simulink model "PositionControlServoValve"  (R2024b)
settings: Solver=daessc  StartTime=0.0  StopTime=4  MaxStep=0.08  RelTol=1e-3  AbsTol=1e-3
PreLoadFcn:
  | PositionControlServoValveInput
values from neighbouring files (symbols this model uses):
  closePosition = 3e-4    (= 0.0003)    [PositionControlServoValveInput.m]
  dampCoeff = 1e-1    (= 0.1)    [PositionControlServoValveInput.m]
  flapperLength = 5e-3    (= 0.005)    [PositionControlServoValveInput.m]
  flapperRotAngle = 3.4928    [PositionControlServoValveInput.m]
  kii = 0.002    [PositionControlServoValveInput.m]
  kip = 0.004    [PositionControlServoValveInput.m]
  kpi = 600    [PositionControlServoValveInput.m]
  kpp = 160    [PositionControlServoValveInput.m]
  kvi = 10    [PositionControlServoValveInput.m]
  kvp = 200    [PositionControlServoValveInput.m]
  motorC = 1    [PositionControlServoValveInput.m]
  motorDampCoeff = 1e-3    (= 0.001)    [PositionControlServoValveInput.m]
  motorR = 750    [PositionControlServoValveInput.m]
  nozCrossSectArea = (pi/4)*(1.6e-3^2)    (= 2.0106192983e-06)    [PositionControlServoValveInput.m]
  overlap = 0.1    [PositionControlServoValveInput.m]
undefined symbols (not defined in the file or in its folder): smiData, X, Y, Z
libraries: fl_lib x174, sm_lib x50, SimscapeFluids_lib x43, nesl_utility x13
(part 4 of 5)

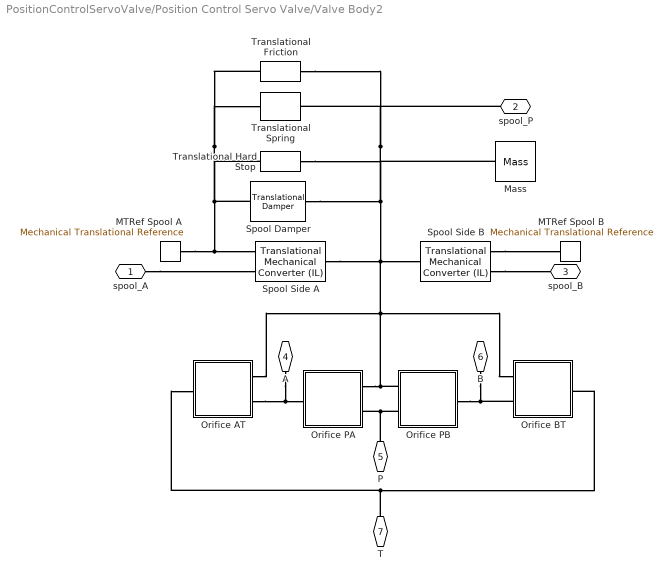
== system PositionControlServoValve/Position Control Servo Valve/Valve Body2 ==
  MTRef Spool A : fl_lib/Mechanical/Translational Elements/Mechanical Translational Reference  Tag=Factory Generic
  MTRef Spool B : fl_lib/Mechanical/Translational Elements/Mechanical Translational Reference  Tag=Factory Generic
  Mass : fl_lib/Mechanical/Translational Elements/Mass  mass=spoolMass kg  num_ports=foundation.enum.numPorts2.one  v_specify=off  v_priority=High  v=0 m/s  v_nominal_specify=off  v_nominal_value=1  v_nominal_unit=m/s  f_specify=off  f_priority=None  f=0 N  f_nominal_specify=off  f_nominal_value=1  f_nominal_unit=N
  Orifice AT : Subsystem  Tag=PublishSubsystem
  Orifice BT : Subsystem
  Orifice PA : Subsystem
  Orifice PB : Subsystem
  Spool Damper : fl_lib/Mechanical/Translational Elements/Translational Damper  Tag=Factory Generic  D=dampCoeff N/(m/s)  v_specify=off  v_priority=High  v=0 m/s  v_nominal_specify=off  v_nominal_value=1  v_nominal_unit=m/s  f_specify=off  f_priority=High  f=0 N  f_nominal_specify=off  f_nominal_value=1  f_nominal_unit=N
  Spool Side A : fl_lib/Isothermal Liquid/Elements/Translational Mechanical Converter (IL)  Tag=Factory Generic  mech_orientation=foundation.enum.MechOrientationTranslational.Positive  displacement_spec=foundation.enum.DisplacementSpec.Calculate  x0=0 m  interface_area=spoolArea mm^2  dead_volume=deadVol m^3  pressure_spec=foundation.enum.pressure_spec.atmospheric  environment_pressure=0.101325 MPa  dynamic_compressibility=simscape.enum.onoff.on  p0=pInitLeftChamber MPa
      settings: InternalSimscapePortConfiguration="{\"Bottom\":[],\"Left\":[{\"id\":\"A\",\"label\":\"A\",\"type\":\"foundation.isothermal_liquid.isothermal_liquid\"},{\"id\":\"C\",\"label\":\"C\",\"type\":\"foundation.mechanical.translational.translational\"}],\"Right\":[{\"id\":\"R\",\"label\":\"R\",\"type\":\"foundation.mechanical.translational.translational\"}],\"Top\":[]}"
  Spool Side B : fl_lib/Isothermal Liquid/Elements/Translational Mechanical Converter (IL)  Tag=Factory Generic  mech_orientation=foundation.enum.MechOrientationTranslational.Negative  displacement_spec=foundation.enum.DisplacementSpec.Calculate  x0=0 m  interface_area=spoolArea mm^2  dead_volume=deadVol m^3  pressure_spec=foundation.enum.pressure_spec.atmospheric  environment_pressure=0.101325 MPa  dynamic_compressibility=simscape.enum.onoff.on  p0=pInitRightChamber MPa
      settings: InternalSimscapePortConfiguration="{\"Bottom\":[],\"Left\":[{\"id\":\"A\",\"label\":\"A\",\"type\":\"foundation.isothermal_liquid.isothermal_liquid\"},{\"id\":\"C\",\"label\":\"C\",\"type\":\"foundation.mechanical.translational.translational\"}],\"Right\":[{\"id\":\"R\",\"label\":\"R\",\"type\":\"foundation.mechanical.translational.translational\"}],\"Top\":[]}"
  Translational Friction : fl_lib/Mechanical/Translational Elements/Translational Friction  brkwy_frc=breakawayF N  brkwy_vel=breakfricV m/s  Col_frc=coloumbF N  visc_coef=dampCoeff N/(m/s)  v_specify=off  v_priority=None  v=0 m/s  v_nominal_specify=off  v_nominal_value=1  v_nominal_unit=m/s  f_specify=off  f_priority=None  f=0 N  f_nominal_specify=off  f_nominal_value=1  f_nominal_unit=N
      settings: InternalSimscapePortConfiguration="{\"Bottom\":[],\"Left\":[{\"id\":\"R\",\"label\":\"R\",\"type\":\"foundation.mechanical.translational.translational\"}],\"Right\":[{\"id\":\"C\",\"label\":\"C\",\"type\":\"foundation.mechanical.translational.translational\"}],\"Top\":[]}"
  Translational Hard Stop : fl_lib/Mechanical/Translational Elements/Translational Hard Stop  upper_bnd=spoolUB mm  lower_bnd=spoolLB mm  model=simscape.enum.hardstop.smooth  stiff_up=hardstopK N/m  stiff_low=hardstopK N/m  D_up=hardstopC N/(m/s)  D_low=hardstopC N/(m/s)  transition=0.1 mm  coeff_rest=0.7  v_tol=0.001 m/s  f_tol=0.001 N  v_specify=off  v_priority=None  v=0 m/s  v_nominal_specify=off  v_nominal_value=1  v_nominal_unit=m/s  f_specify=off  f_priority=None  f=0 N  f_nominal_specify=off  f_nominal_value=1  f_nominal_unit=N  x_specify=off  x_priority=High  x=0 m  x_nominal_specify=off  x_nominal_value=1  x_nominal_unit=m  M_specify=off  M_priority=None  M=0
  Translational Spring : fl_lib/Mechanical/Translational Elements/Translational Spring  spr_rate=springCoeff N/m  v_specify=off  v_priority=None  v=0 m/s  v_nominal_specify=off  v_nominal_value=1  v_nominal_unit=m/s  f_specify=off  f_priority=None  f=0 N  f_nominal_specify=off  f_nominal_value=1  f_nominal_unit=N  x_specify=off  x_priority=High  x=0 m  x_nominal_specify=off  x_nominal_value=1  x_nominal_unit=m
  spool_A : PMIOPort  Side=Left
  spool_P : PMIOPort  Port=2  Side=Left
  spool_B : PMIOPort  Port=3  Side=Left
  A : PMIOPort  Port=4  Side=Right
  P : PMIOPort  Port=5  Side=Right
  B : PMIOPort  Port=6  Side=Right
  T : PMIOPort  Port=7  Side=Right
  connections:
  A/RConn1 -- Orifice AT/LConn2 -- Orifice PA/RConn1
  P/RConn1 -- Orifice PB/LConn2 -- Orifice PA/LConn2
  Orifice BT/LConn2 -- B/RConn1 -- Orifice PB/RConn1
  T/RConn1 -- Orifice BT/RConn1 -- Orifice AT/RConn1
  Spool Side B/LConn2 -- MTRef Spool B/LConn1
  Spool Side B/LConn1 -- spool_B/RConn1
  Orifice PB/LConn1 -- Orifice PA/LConn1 -- Orifice BT/LConn1 -- Spool Side B/RConn1 -- Mass/LConn1 -- spool_P/RConn1 -- Translational Friction/LConn1 -- Translational Spring/LConn1 -- Translational Hard Stop/LConn1 -- Spool Damper/LConn1 -- Spool Side A/RConn1 -- Orifice AT/LConn1
  spool_A/RConn1 -- Spool Side A/LConn1
  Spool Damper/RConn1 -- Translational Hard Stop/RConn1 -- Translational Friction/RConn1 -- Translational Spring/RConn1 -- MTRef Spool A/LConn1 -- Spool Side A/LConn2

== system PositionControlServoValve/Servo Controller/Current controller ==
  Target Current : Inport
  Motor Current : Inport  Port=2
  Add1 : Sum  Inputs=+-
  Add2 : Sum
  Gain1 : Gain  Gain=kip
  Gain2 : Gain  Gain=kii
  Integrator Limited : Integrator  LimitOutput=on
  Saturation : Saturate  UpperLimit=1  LowerLimit=-1
  PWM ref : Outport
  wires:
  Target Current/1 -> Add1/1
  Motor Current/1 -> Add1/2
  Gain1/1 -> Add2/1
  Integrator Limited/1 -> Add2/2
  Gain2/1 -> Integrator Limited/1
  Add1/1 -> Gain1/1, Gain2/1
  Add2/1 -> Saturation/1
  Saturation/1 -> PWM ref/1

== system PositionControlServoValve/Servo Controller/Current controller1 ==
  Target Current : Inport
  Motor Current : Inport  Port=2
  Add1 : Sum  Inputs=+-
  Add2 : Sum
  Gain1 : Gain  Gain=kip
  Gain2 : Gain  Gain=kii
  Integrator Limited : Integrator  LimitOutput=on
  Saturation : Saturate  UpperLimit=1  LowerLimit=-1
  PWM ref : Outport
  wires:
  Target Current/1 -> Add1/1
  Motor Current/1 -> Add1/2
  Gain1/1 -> Add2/1
  Integrator Limited/1 -> Add2/2
  Gain2/1 -> Integrator Limited/1
  Add1/1 -> Gain1/1, Gain2/1
  Add2/1 -> Saturation/1
  Saturation/1 -> PWM ref/1

== system PositionControlServoValve/Servo Controller/Current controller2 ==
  Target Current : Inport
  Motor Current : Inport  Port=2
  Add1 : Sum  Inputs=+-
  Add2 : Sum
  Gain1 : Gain  Gain=kip
  Gain2 : Gain  Gain=kii
  Integrator Limited : Integrator  LimitOutput=on
  Saturation : Saturate  UpperLimit=1  LowerLimit=-1
  PWM ref : Outport
  wires:
  Target Current/1 -> Add1/1
  Motor Current/1 -> Add1/2
  Gain1/1 -> Add2/1
  Integrator Limited/1 -> Add2/2
  Gain2/1 -> Integrator Limited/1
  Add1/1 -> Gain1/1, Gain2/1
  Add2/1 -> Saturation/1
  Saturation/1 -> PWM ref/1

== system PositionControlServoValve/Servo Controller/Position controller ==
  Target Position : Inport
  Actuator Position : Inport  Port=2
  Add : Sum  Inputs=+-
  Add2 : Sum
  Gain : Gain
  Gain1 : Gain  Gain=kpp
  Gain2 : Gain  Gain=kpi
  Integrator Limited : Integrator  LimitOutput=on
  Target velocity : Outport
  wires:
  Target Position/1 -> Add/1
  Actuator Position/1 -> Add/2
  Gain2/1 -> Integrator Limited/1
  Gain1/1 -> Add2/1
  Integrator Limited/1 -> Add2/2
  Add/1 -> Gain/1
  Add2/1 -> Target velocity/1
  Gain/1 -> Gain1/1, Gain2/1

== system PositionControlServoValve/Servo Controller/Position controller1 ==
  Target Position : Inport
  Actuator Position : Inport  Port=2
  Add : Sum  Inputs=+-
  Add2 : Sum
  Gain : Gain
  Gain1 : Gain  Gain=kpp
  Gain2 : Gain  Gain=kpi
  Integrator Limited : Integrator  LimitOutput=on
  Target velocity : Outport
  wires:
  Target Position/1 -> Add/1
  Actuator Position/1 -> Add/2
  Gain2/1 -> Integrator Limited/1
  Gain1/1 -> Add2/1
  Integrator Limited/1 -> Add2/2
  Add/1 -> Gain/1
  Add2/1 -> Target velocity/1
  Gain/1 -> Gain1/1, Gain2/1

== system PositionControlServoValve/Servo Controller/Position controller2 ==
  Target Position : Inport
  Actuator Position : Inport  Port=2
  Add : Sum  Inputs=+-
  Add2 : Sum
  Gain : Gain
  Gain1 : Gain  Gain=kpp
  Gain2 : Gain  Gain=kpi
  Integrator Limited : Integrator  LimitOutput=on
  Target velocity : Outport
  wires:
  Target Position/1 -> Add/1
  Actuator Position/1 -> Add/2
  Gain2/1 -> Integrator Limited/1
  Gain1/1 -> Add2/1
  Integrator Limited/1 -> Add2/2
  Add/1 -> Gain/1
  Add2/1 -> Target velocity/1
  Gain/1 -> Gain1/1, Gain2/1

== system PositionControlServoValve/Servo Controller/Velocity controller ==
  Target Velocity : Inport
  Actuator Velocity : Inport  Port=2
  Add : Sum  Inputs=+-
  Add2 : Sum
  Gain : Gain  Gain=-1
  Gain1 : Gain  Gain=kvp
  Gain2 : Gain  Gain=kvi
  Integrator Limited : Integrator  LimitOutput=on
  Target Current : Outport
  wires:
  Target Velocity/1 -> Add/1
  Actuator Velocity/1 -> Add/2
  Add/1 -> Gain/1
  Add2/1 -> Target Current/1
  Gain1/1 -> Add2/1
  Integrator Limited/1 -> Add2/2
  Gain2/1 -> Integrator Limited/1
  Gain/1 -> Gain2/1, Gain1/1

== system PositionControlServoValve/Servo Controller/Velocity controller1 ==
  Target Velocity : Inport
  Actuator Velocity : Inport  Port=2
  Add : Sum  Inputs=+-
  Add2 : Sum
  Gain : Gain  Gain=-1
  Gain1 : Gain  Gain=kvp
  Gain2 : Gain  Gain=kvi
  Integrator Limited : Integrator  LimitOutput=on
  Target Current : Outport
  wires:
  Target Velocity/1 -> Add/1
  Actuator Velocity/1 -> Add/2
  Add/1 -> Gain/1
  Add2/1 -> Target Current/1
  Gain1/1 -> Add2/1
  Integrator Limited/1 -> Add2/2
  Gain2/1 -> Integrator Limited/1
  Gain/1 -> Gain2/1, Gain1/1

== system PositionControlServoValve/Servo Controller/Velocity controller2 ==
  Target Velocity : Inport
  Actuator Velocity : Inport  Port=2
  Add : Sum  Inputs=+-
  Add2 : Sum
  Gain : Gain  Gain=-1
  Gain1 : Gain  Gain=kvp
  Gain2 : Gain  Gain=kvi
  Integrator Limited : Integrator  LimitOutput=on
  Target Current : Outport
  wires:
  Target Velocity/1 -> Add/1
  Actuator Velocity/1 -> Add/2
  Add/1 -> Gain/1
  Add2/1 -> Target Current/1
  Gain1/1 -> Add2/1
  Integrator Limited/1 -> Add2/2
  Gain2/1 -> Integrator Limited/1
  Gain/1 -> Gain2/1, Gain1/1

== system PositionControlServoValve/Position Control Servo Valve/Torque Motor With Flapper/Current sensor ==
  Current Sensor : fl_lib/Electrical/Electrical Sensors/Current Sensor
  Current FEM : nesl_utility/PS-Simulink Converter  PhysicalDomain=network_engine_domain  SubClassName=ps_output  LeftPortType=input  RightPortType=output  PseudoPeriodic=off  Frequencies=[]  VectorFormat=1-D array  Unit=mA  AffineConversion=off
  + : PMIOPort  Side=Left
  - : PMIOPort  Port=2  Side=Right
  motorCurrent : Outport
  wires:
  Current FEM/1 -> motorCurrent/1
  connections:
  Current Sensor/RConn1 -- Current FEM/LConn1
  Current Sensor/RConn2 -- -/RConn1
  +/RConn1 -- Current Sensor/LConn1

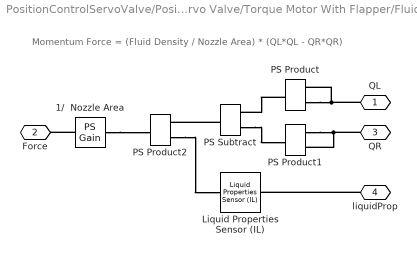
== system PositionControlServoValve/Position Control Servo Valve/Torque Motor With Flapper/Fluid Momentum Force ==
  note: Momentum Force = (Fluid Density / Nozzle Area) * (QL*QL - QR*QR)
  1/  Nozzle Area : fl_lib/Physical Signals/Functions/PS Gain  gain=1/nozCrossSectArea 1/m^2
  Liquid Properties Sensor (IL) : fl_lib/Isothermal Liquid/Sensors/Liquid Properties Sensor (IL)  density_measure=simscape.enum.onoff.on  bulk_modulus_measure=simscape.enum.onoff.off  entrained_air_measure=simscape.enum.onoff.off
      settings: InternalSimscapePortConfiguration="{\"Bottom\":[],\"Left\":[{\"id\":\"A\",\"label\":\"A\",\"type\":\"foundation.isothermal_liquid.isothermal_liquid\"}],\"Right\":[{\"id\":\"rho\",\"label\":\"rho\",\"type\":\"output\"}],\"Top\":[]}"
  PS Product : fl_lib/Physical Signals/Functions/PS Product
  PS Product1 : fl_lib/Physical Signals/Functions/PS Product
  PS Product2 : fl_lib/Physical Signals/Functions/PS Product
  PS Subtract : fl_lib/Physical Signals/Functions/PS Subtract
  QL : PMIOPort  Side=Right
  Force : PMIOPort  Port=2  Side=Left
  QR : PMIOPort  Port=3  Side=Right
  liquidProp : PMIOPort  Port=4  Side=Right
  connections:
  PS Product/LConn2 -- QL/RConn1 -- PS Product/LConn1
  PS Product1/LConn1 -- QR/RConn1 -- PS Product1/LConn2
  PS Product/RConn1 -- PS Subtract/LConn1
  1/  Nozzle Area/LConn1 -- PS Product2/RConn1
  1/  Nozzle Area/RConn1 -- Force/RConn1
  PS Subtract/RConn1 -- PS Product2/LConn1
  PS Subtract/LConn2 -- PS Product1/RConn1
  liquidProp/RConn1 -- Liquid Properties Sensor (IL)/LConn1
  PS Product2/LConn2 -- Liquid Properties Sensor (IL)/RConn1

== system PositionControlServoValve/Position Control Servo Valve/Torque Motor With Flapper/PWM drive ==
  PWM : Inport
  Controlled Voltage Source : fl_lib/Electrical/Electrical Sources/Controlled Voltage Source
  DC supply : fl_lib/Physical Signals/Functions/PS Gain  gain=12 V
  ERef1 : fl_lib/Electrical/Electrical Elements/Electrical Reference
  Simulink-PS Converter : nesl_utility/Simulink-PS Converter  PhysicalDomain=network_engine_domain  SubClassName=ps_input  LeftPortType=input  RightPortType=output  PseudoPeriodic=off  Frequencies=[]  NoiseDistribution=none  NoiseParameters=[]  Unit=1  AffineConversion=off  FilteringAndDerivatives=filter  SimscapeFilterOrder=1  InputFilterTimeConstant=0.0001  UdotUserProvided=1
  V : PMIOPort  Side=Right
  wires:
  PWM/1 -> Simulink-PS Converter/1
  connections:
  Simulink-PS Converter/RConn1 -- DC supply/LConn1
  ERef1/LConn1 -- Controlled Voltage Source/RConn2
  V/RConn1 -- Controlled Voltage Source/LConn1
  DC supply/RConn1 -- Controlled Voltage Source/RConn1

== system PositionControlServoValve/Position Control Servo Valve/Torque Motor With Flapper/Position Sensor ==
  Ideal Translational Motion Sensor : fl_lib/Mechanical/Mechanical Sensors/Ideal Translational Motion Sensor  reference=foundation.enum.MeasurementReference.difference  acceleration_port=false  velocity_port=true  position_port=true  offset=0 m
  Mechanical Translational Reference : fl_lib/Mechanical/Translational Elements/Mechanical Translational Reference
  R : PMIOPort  Side=Left
  P : PMIOPort  Port=2  Side=Right
  connections:
  Ideal Translational Motion Sensor/LConn1 -- R/RConn1
  Ideal Translational Motion Sensor/RConn3 -- P/RConn1
  Mechanical Translational Reference/LConn1 -- Ideal Translational Motion Sensor/RConn1

== system PositionControlServoValve/Position Control Servo Valve/Torque Motor With Flapper/Torque Motor ==
  Hard Stop : fl_lib/Mechanical/Rotational Elements/Rotational Hard Stop  upper_bnd=flapperRotAngle deg  lower_bnd=-flapperRotAngle deg  model=simscape.enum.hardstop.smooth  stiff_up=1e+7 N*m/rad  stiff_low=1e+7 N*m/rad  D_up=1e6 N*m/(rad/s)  D_low=1e6 N*m/(rad/s)  transition=0.001 rad  coeff_rest=0.7  w_tol=0.1 rad/s  trq_tol=0.001 N*m  w_specify=off  w_priority=High  w=0 rad/s  w_nominal_specify=off  w_nominal_value=1  w_nominal_unit=rad/s  t_specify=off  t_priority=High  t=0 N*m  t_nominal_specify=off  t_nominal_value=1  t_nominal_unit=N*m  phi_specify=on  phi_priority=High  phi=0 deg  phi_nominal_specify=off  phi_nominal_value=1  phi_nominal_unit=rad  M_specify=off  M_priority=None  M=0
  Inductor : fl_lib/Electrical/Electrical Elements/Inductor  l=motorI mH  r=0 Ohm  g=1e-9 1/Ohm  i_specify=off  i_priority=High  i=0 A  i_nominal_specify=off  i_nominal_value=1  i_nominal_unit=A  v_specify=off  v_priority=High  v=0 V  v_nominal_specify=off  v_nominal_value=1  v_nominal_unit=V  i_L_specify=on  i_L_priority=High  i_L=0 A  i_L_nominal_specify=off  i_L_nominal_value=1  i_L_nominal_unit=A
  Inertia : fl_lib/Mechanical/Rotational Elements/Inertia  inertia=motorInertia mm^2*g  num_ports=foundation.enum.numPorts2.one  w_specify=on  w_priority=High  w=0 rad/s  w_nominal_specify=off  w_nominal_value=1  w_nominal_unit=rad/s  t_specify=off  t_priority=High  t=0 N*m  t_nominal_specify=off  t_nominal_value=1  t_nominal_unit=N*m
  Resistor : fl_lib/Electrical/Electrical Elements/Resistor  R=motorR Ohm  i_specify=off  i_priority=High  i=0 A  i_nominal_specify=off  i_nominal_value=1  i_nominal_unit=A  v_specify=off  v_priority=High  v=0 V  v_nominal_specify=off  v_nominal_value=1  v_nominal_unit=V
  Rotational Electromechanical Converter : fl_lib/Electrical/Electrical Elements/Rotational Electromechanical Converter  K=motorC V/(rad/s)  i_specify=on  i_priority=High  i=0 A  i_nominal_specify=off  i_nominal_value=1  i_nominal_unit=A  v_specify=off  v_priority=High  v=0 V  v_nominal_specify=off  v_nominal_value=1  v_nominal_unit=V  t_specify=off  t_priority=High  t=0 N*m  t_nominal_specify=off  t_nominal_value=1  t_nominal_unit=N*m  w_specify=off  w_priority=None  w=0 rad/s  w_nominal_specify=off  w_nominal_value=1  w_nominal_unit=rad/s
  + : PMIOPort  Side=Left
  R : PMIOPort  Port=2  Side=Left
  - : PMIOPort  Port=3  Side=Right
  C : PMIOPort  Port=4  Side=Right
  connections:
  C/RConn1 -- Rotational Electromechanical Converter/RConn2 -- Hard Stop/RConn1
  -/RConn1 -- Resistor/LConn1
  Resistor/RConn1 -- Rotational Electromechanical Converter/RConn1
  Hard Stop/LConn1 -- R/RConn1 -- Rotational Electromechanical Converter/LConn2 -- Inertia/LConn1
  +/RConn1 -- Inductor/LConn1
  Inductor/RConn1 -- Rotational Electromechanical Converter/LConn1

== system PositionControlServoValve/Position Control Servo Valve/Torque Motor With Flapper1/Current sensor ==
  Current Sensor : fl_lib/Electrical/Electrical Sensors/Current Sensor
  Current FEM : nesl_utility/PS-Simulink Converter  PhysicalDomain=network_engine_domain  SubClassName=ps_output  LeftPortType=input  RightPortType=output  PseudoPeriodic=off  Frequencies=[]  VectorFormat=1-D array  Unit=mA  AffineConversion=off
  + : PMIOPort  Side=Left
  - : PMIOPort  Port=2  Side=Right
  motorCurrent : Outport
  wires:
  Current FEM/1 -> motorCurrent/1
  connections:
  Current Sensor/RConn1 -- Current FEM/LConn1
  Current Sensor/RConn2 -- -/RConn1
  +/RConn1 -- Current Sensor/LConn1

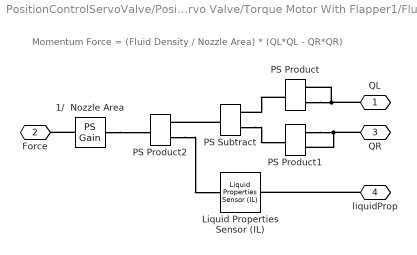
== system PositionControlServoValve/Position Control Servo Valve/Torque Motor With Flapper1/Fluid Momentum Force ==
  note: Momentum Force = (Fluid Density / Nozzle Area) * (QL*QL - QR*QR)
  1/  Nozzle Area : fl_lib/Physical Signals/Functions/PS Gain  gain=1/nozCrossSectArea 1/m^2
  Liquid Properties Sensor (IL) : fl_lib/Isothermal Liquid/Sensors/Liquid Properties Sensor (IL)  density_measure=simscape.enum.onoff.on  bulk_modulus_measure=simscape.enum.onoff.off  entrained_air_measure=simscape.enum.onoff.off
      settings: InternalSimscapePortConfiguration="{\"Bottom\":[],\"Left\":[{\"id\":\"A\",\"label\":\"A\",\"type\":\"foundation.isothermal_liquid.isothermal_liquid\"}],\"Right\":[{\"id\":\"rho\",\"label\":\"rho\",\"type\":\"output\"}],\"Top\":[]}"
  PS Product : fl_lib/Physical Signals/Functions/PS Product
  PS Product1 : fl_lib/Physical Signals/Functions/PS Product
  PS Product2 : fl_lib/Physical Signals/Functions/PS Product
  PS Subtract : fl_lib/Physical Signals/Functions/PS Subtract
  QL : PMIOPort  Side=Right
  Force : PMIOPort  Port=2  Side=Left
  QR : PMIOPort  Port=3  Side=Right
  liquidProp : PMIOPort  Port=4  Side=Right
  connections:
  PS Product/LConn2 -- QL/RConn1 -- PS Product/LConn1
  PS Product1/LConn1 -- QR/RConn1 -- PS Product1/LConn2
  PS Product/RConn1 -- PS Subtract/LConn1
  1/  Nozzle Area/LConn1 -- PS Product2/RConn1
  1/  Nozzle Area/RConn1 -- Force/RConn1
  PS Subtract/RConn1 -- PS Product2/LConn1
  PS Subtract/LConn2 -- PS Product1/RConn1
  liquidProp/RConn1 -- Liquid Properties Sensor (IL)/LConn1
  PS Product2/LConn2 -- Liquid Properties Sensor (IL)/RConn1

== system PositionControlServoValve/Position Control Servo Valve/Torque Motor With Flapper1/PWM drive ==
  PWM : Inport
  Controlled Voltage Source : fl_lib/Electrical/Electrical Sources/Controlled Voltage Source
  DC supply : fl_lib/Physical Signals/Functions/PS Gain  gain=12 V
  ERef1 : fl_lib/Electrical/Electrical Elements/Electrical Reference
  Simulink-PS Converter : nesl_utility/Simulink-PS Converter  PhysicalDomain=network_engine_domain  SubClassName=ps_input  LeftPortType=input  RightPortType=output  PseudoPeriodic=off  Frequencies=[]  NoiseDistribution=none  NoiseParameters=[]  Unit=1  AffineConversion=off  FilteringAndDerivatives=filter  SimscapeFilterOrder=1  InputFilterTimeConstant=0.0001  UdotUserProvided=1
  V : PMIOPort  Side=Right
  wires:
  PWM/1 -> Simulink-PS Converter/1
  connections:
  Simulink-PS Converter/RConn1 -- DC supply/LConn1
  ERef1/LConn1 -- Controlled Voltage Source/RConn2
  V/RConn1 -- Controlled Voltage Source/LConn1
  DC supply/RConn1 -- Controlled Voltage Source/RConn1

== system PositionControlServoValve/Position Control Servo Valve/Torque Motor With Flapper1/Position Sensor ==
  Ideal Translational Motion Sensor : fl_lib/Mechanical/Mechanical Sensors/Ideal Translational Motion Sensor  reference=foundation.enum.MeasurementReference.difference  acceleration_port=false  velocity_port=true  position_port=true  offset=0 m
  Mechanical Translational Reference : fl_lib/Mechanical/Translational Elements/Mechanical Translational Reference
  R : PMIOPort  Side=Left
  P : PMIOPort  Port=2  Side=Right
  connections:
  Ideal Translational Motion Sensor/LConn1 -- R/RConn1
  Ideal Translational Motion Sensor/RConn3 -- P/RConn1
  Mechanical Translational Reference/LConn1 -- Ideal Translational Motion Sensor/RConn1

== system PositionControlServoValve/Position Control Servo Valve/Torque Motor With Flapper1/Torque Motor ==
  Hard Stop : fl_lib/Mechanical/Rotational Elements/Rotational Hard Stop  upper_bnd=flapperRotAngle deg  lower_bnd=-flapperRotAngle deg  model=simscape.enum.hardstop.smooth  stiff_up=1e+7 N*m/rad  stiff_low=1e+7 N*m/rad  D_up=1e6 N*m/(rad/s)  D_low=1e6 N*m/(rad/s)  transition=0.001 rad  coeff_rest=0.7  w_tol=0.1 rad/s  trq_tol=0.001 N*m  w_specify=off  w_priority=High  w=0 rad/s  w_nominal_specify=off  w_nominal_value=1  w_nominal_unit=rad/s  t_specify=off  t_priority=High  t=0 N*m  t_nominal_specify=off  t_nominal_value=1  t_nominal_unit=N*m  phi_specify=on  phi_priority=High  phi=0 deg  phi_nominal_specify=off  phi_nominal_value=1  phi_nominal_unit=rad  M_specify=off  M_priority=None  M=0
  Inductor : fl_lib/Electrical/Electrical Elements/Inductor  l=motorI mH  r=0 Ohm  g=1e-9 1/Ohm  i_specify=off  i_priority=High  i=0 A  i_nominal_specify=off  i_nominal_value=1  i_nominal_unit=A  v_specify=off  v_priority=High  v=0 V  v_nominal_specify=off  v_nominal_value=1  v_nominal_unit=V  i_L_specify=on  i_L_priority=High  i_L=0 A  i_L_nominal_specify=off  i_L_nominal_value=1  i_L_nominal_unit=A
  Inertia : fl_lib/Mechanical/Rotational Elements/Inertia  inertia=motorInertia mm^2*g  num_ports=foundation.enum.numPorts2.one  w_specify=on  w_priority=High  w=0 rad/s  w_nominal_specify=off  w_nominal_value=1  w_nominal_unit=rad/s  t_specify=off  t_priority=High  t=0 N*m  t_nominal_specify=off  t_nominal_value=1  t_nominal_unit=N*m
  Resistor : fl_lib/Electrical/Electrical Elements/Resistor  R=motorR Ohm  i_specify=off  i_priority=High  i=0 A  i_nominal_specify=off  i_nominal_value=1  i_nominal_unit=A  v_specify=off  v_priority=High  v=0 V  v_nominal_specify=off  v_nominal_value=1  v_nominal_unit=V
  Rotational Electromechanical Converter : fl_lib/Electrical/Electrical Elements/Rotational Electromechanical Converter  K=motorC V/(rad/s)  i_specify=on  i_priority=High  i=0 A  i_nominal_specify=off  i_nominal_value=1  i_nominal_unit=A  v_specify=off  v_priority=High  v=0 V  v_nominal_specify=off  v_nominal_value=1  v_nominal_unit=V  t_specify=off  t_priority=High  t=0 N*m  t_nominal_specify=off  t_nominal_value=1  t_nominal_unit=N*m  w_specify=off  w_priority=None  w=0 rad/s  w_nominal_specify=off  w_nominal_value=1  w_nominal_unit=rad/s
  + : PMIOPort  Side=Left
  R : PMIOPort  Port=2  Side=Left
  - : PMIOPort  Port=3  Side=Right
  C : PMIOPort  Port=4  Side=Right
  connections:
  C/RConn1 -- Rotational Electromechanical Converter/RConn2 -- Hard Stop/RConn1
  -/RConn1 -- Resistor/LConn1
  Resistor/RConn1 -- Rotational Electromechanical Converter/RConn1
  Hard Stop/LConn1 -- R/RConn1 -- Rotational Electromechanical Converter/LConn2 -- Inertia/LConn1
  +/RConn1 -- Inductor/LConn1
  Inductor/RConn1 -- Rotational Electromechanical Converter/LConn1

== system PositionControlServoValve/Position Control Servo Valve/Torque Motor With Flapper2/Current sensor ==
  Current Sensor : fl_lib/Electrical/Electrical Sensors/Current Sensor
  Current FEM : nesl_utility/PS-Simulink Converter  PhysicalDomain=network_engine_domain  SubClassName=ps_output  LeftPortType=input  RightPortType=output  PseudoPeriodic=off  Frequencies=[]  VectorFormat=1-D array  Unit=mA  AffineConversion=off
  + : PMIOPort  Side=Left
  - : PMIOPort  Port=2  Side=Right
  motorCurrent : Outport
  wires:
  Current FEM/1 -> motorCurrent/1
  connections:
  Current Sensor/RConn1 -- Current FEM/LConn1
  Current Sensor/RConn2 -- -/RConn1
  +/RConn1 -- Current Sensor/LConn1

== system PositionControlServoValve/Position Control Servo Valve/Torque Motor With Flapper2/Fluid Momentum Force ==
  note: Momentum Force = (Fluid Density / Nozzle Area) * (QL*QL - QR*QR)
  1/  Nozzle Area : fl_lib/Physical Signals/Functions/PS Gain  gain=1/nozCrossSectArea 1/m^2
  Liquid Properties Sensor (IL) : fl_lib/Isothermal Liquid/Sensors/Liquid Properties Sensor (IL)  density_measure=simscape.enum.onoff.on  bulk_modulus_measure=simscape.enum.onoff.off  entrained_air_measure=simscape.enum.onoff.off
      settings: InternalSimscapePortConfiguration="{\"Bottom\":[],\"Left\":[{\"id\":\"A\",\"label\":\"A\",\"type\":\"foundation.isothermal_liquid.isothermal_liquid\"}],\"Right\":[{\"id\":\"rho\",\"label\":\"rho\",\"type\":\"output\"}],\"Top\":[]}"
  PS Product : fl_lib/Physical Signals/Functions/PS Product
  PS Product1 : fl_lib/Physical Signals/Functions/PS Product
  PS Product2 : fl_lib/Physical Signals/Functions/PS Product
  PS Subtract : fl_lib/Physical Signals/Functions/PS Subtract
  QL : PMIOPort  Side=Right
  Force : PMIOPort  Port=2  Side=Left
  QR : PMIOPort  Port=3  Side=Right
  liquidProp : PMIOPort  Port=4  Side=Right
  connections:
  PS Product/LConn2 -- QL/RConn1 -- PS Product/LConn1
  PS Product1/LConn1 -- QR/RConn1 -- PS Product1/LConn2
  PS Product/RConn1 -- PS Subtract/LConn1
  1/  Nozzle Area/LConn1 -- PS Product2/RConn1
  1/  Nozzle Area/RConn1 -- Force/RConn1
  PS Subtract/RConn1 -- PS Product2/LConn1
  PS Subtract/LConn2 -- PS Product1/RConn1
  liquidProp/RConn1 -- Liquid Properties Sensor (IL)/LConn1
  PS Product2/LConn2 -- Liquid Properties Sensor (IL)/RConn1

== system PositionControlServoValve/Position Control Servo Valve/Torque Motor With Flapper2/PWM drive ==
  PWM : Inport
  Controlled Voltage Source : fl_lib/Electrical/Electrical Sources/Controlled Voltage Source
  DC supply : fl_lib/Physical Signals/Functions/PS Gain  gain=12 V
  ERef1 : fl_lib/Electrical/Electrical Elements/Electrical Reference
  Simulink-PS Converter : nesl_utility/Simulink-PS Converter  PhysicalDomain=network_engine_domain  SubClassName=ps_input  LeftPortType=input  RightPortType=output  PseudoPeriodic=off  Frequencies=[]  NoiseDistribution=none  NoiseParameters=[]  Unit=1  AffineConversion=off  FilteringAndDerivatives=filter  SimscapeFilterOrder=1  InputFilterTimeConstant=0.0001  UdotUserProvided=1
  V : PMIOPort  Side=Right
  wires:
  PWM/1 -> Simulink-PS Converter/1
  connections:
  Simulink-PS Converter/RConn1 -- DC supply/LConn1
  ERef1/LConn1 -- Controlled Voltage Source/RConn2
  V/RConn1 -- Controlled Voltage Source/LConn1
  DC supply/RConn1 -- Controlled Voltage Source/RConn1

== system PositionControlServoValve/Position Control Servo Valve/Torque Motor With Flapper2/Position Sensor ==
  Ideal Translational Motion Sensor : fl_lib/Mechanical/Mechanical Sensors/Ideal Translational Motion Sensor  reference=foundation.enum.MeasurementReference.difference  acceleration_port=false  velocity_port=true  position_port=true  offset=0 m
  Mechanical Translational Reference : fl_lib/Mechanical/Translational Elements/Mechanical Translational Reference
  R : PMIOPort  Side=Left
  P : PMIOPort  Port=2  Side=Right
  connections:
  Ideal Translational Motion Sensor/LConn1 -- R/RConn1
  Ideal Translational Motion Sensor/RConn3 -- P/RConn1
  Mechanical Translational Reference/LConn1 -- Ideal Translational Motion Sensor/RConn1

== system PositionControlServoValve/Position Control Servo Valve/Torque Motor With Flapper2/Torque Motor ==
  Hard Stop : fl_lib/Mechanical/Rotational Elements/Rotational Hard Stop  upper_bnd=flapperRotAngle deg  lower_bnd=-flapperRotAngle deg  model=simscape.enum.hardstop.smooth  stiff_up=1e+7 N*m/rad  stiff_low=1e+7 N*m/rad  D_up=1e6 N*m/(rad/s)  D_low=1e6 N*m/(rad/s)  transition=0.001 rad  coeff_rest=0.7  w_tol=0.1 rad/s  trq_tol=0.001 N*m  w_specify=off  w_priority=High  w=0 rad/s  w_nominal_specify=off  w_nominal_value=1  w_nominal_unit=rad/s  t_specify=off  t_priority=High  t=0 N*m  t_nominal_specify=off  t_nominal_value=1  t_nominal_unit=N*m  phi_specify=on  phi_priority=High  phi=0 deg  phi_nominal_specify=off  phi_nominal_value=1  phi_nominal_unit=rad  M_specify=off  M_priority=None  M=0
  Inductor : fl_lib/Electrical/Electrical Elements/Inductor  l=motorI mH  r=0 Ohm  g=1e-9 1/Ohm  i_specify=off  i_priority=High  i=0 A  i_nominal_specify=off  i_nominal_value=1  i_nominal_unit=A  v_specify=off  v_priority=High  v=0 V  v_nominal_specify=off  v_nominal_value=1  v_nominal_unit=V  i_L_specify=on  i_L_priority=High  i_L=0 A  i_L_nominal_specify=off  i_L_nominal_value=1  i_L_nominal_unit=A
  Inertia : fl_lib/Mechanical/Rotational Elements/Inertia  inertia=motorInertia mm^2*g  num_ports=foundation.enum.numPorts2.one  w_specify=on  w_priority=High  w=0 rad/s  w_nominal_specify=off  w_nominal_value=1  w_nominal_unit=rad/s  t_specify=off  t_priority=High  t=0 N*m  t_nominal_specify=off  t_nominal_value=1  t_nominal_unit=N*m
  Resistor : fl_lib/Electrical/Electrical Elements/Resistor  R=motorR Ohm  i_specify=off  i_priority=High  i=0 A  i_nominal_specify=off  i_nominal_value=1  i_nominal_unit=A  v_specify=off  v_priority=High  v=0 V  v_nominal_specify=off  v_nominal_value=1  v_nominal_unit=V
  Rotational Electromechanical Converter : fl_lib/Electrical/Electrical Elements/Rotational Electromechanical Converter  K=motorC V/(rad/s)  i_specify=on  i_priority=High  i=0 A  i_nominal_specify=off  i_nominal_value=1  i_nominal_unit=A  v_specify=off  v_priority=High  v=0 V  v_nominal_specify=off  v_nominal_value=1  v_nominal_unit=V  t_specify=off  t_priority=High  t=0 N*m  t_nominal_specify=off  t_nominal_value=1  t_nominal_unit=N*m  w_specify=off  w_priority=None  w=0 rad/s  w_nominal_specify=off  w_nominal_value=1  w_nominal_unit=rad/s
  + : PMIOPort  Side=Left
  R : PMIOPort  Port=2  Side=Left
  - : PMIOPort  Port=3  Side=Right
  C : PMIOPort  Port=4  Side=Right
  connections:
  C/RConn1 -- Rotational Electromechanical Converter/RConn2 -- Hard Stop/RConn1
  -/RConn1 -- Resistor/LConn1
  Resistor/RConn1 -- Rotational Electromechanical Converter/RConn1
  Hard Stop/LConn1 -- R/RConn1 -- Rotational Electromechanical Converter/LConn2 -- Inertia/LConn1
  +/RConn1 -- Inductor/LConn1
  Inductor/RConn1 -- Rotational Electromechanical Converter/LConn1

== system PositionControlServoValve/Position Control Servo Valve/Valve Body/Orifice AT ==
  Hydraulic Force : fl_lib/Mechanical/Mechanical Sources/Ideal Force Source  Tag=Factory Generic
  MTRef Force : fl_lib/Mechanical/Translational Elements/Mechanical Translational Reference  Tag=Factory Generic
  MTRef Sensor : fl_lib/Mechanical/Translational Elements/Mechanical Translational Reference  Tag=Factory Generic
  Motion Sensor : fl_lib/Mechanical/Mechanical Sensors/Ideal Translational Motion Sensor  Tag=Factory Generic  reference=foundation.enum.MeasurementReference.difference  acceleration_port=false  velocity_port=true  position_port=true  offset=0 m
  Orifice : SimscapeFluids_lib/Isothermal Liquid/Valves & Orifices/Orifices/Spool Orifice (IL)  Tag=Factory Generic  orifice_spec=fluids.isothermal_liquid.valves_orifices.orifices.enum.spool_orifice.rectangle_slot  diameter_hole=5e-3 m  num_hole=6  width=orificeWidth mm  del_S_max="spoolTravel  mm"  S_min=-overlap mm  open_orientation=fluids.isothermal_liquid.valves_orifices.enum.spool_orientation.negative  flow_force_spec=simscape.enum.onoff.off  clearance=1e-5 m  area_leak=1e-9 m^2  area=inf m^2  Cd=0.7  Re_c=150  smoothing_factor=0  pressure_recovery=simscape.enum.onoff.off
      settings: InternalSimscapePortConfiguration="{\"Bottom\":[],\"Left\":[{\"id\":\"S\",\"label\":\"S\",\"type\":\"input\"},{\"id\":\"A\",\"label\":\"A\",\"type\":\"foundation.isothermal_liquid.isothermal_liquid\"}],\"Right\":[{\"id\":\"B\",\"label\":\"B\",\"type\":\"foundation.isothermal_liquid.isothermal_liquid\"}],\"Top\":[]}"
  Spool Orifice Hydraulic Force : SimscapeFluids_lib/Isothermal Liquid/Valves & Orifices/Valve Actuators & Forces/Spool Orifice Flow Force (IL)  orifice_spec=fluids.isothermal_liquid.valves_orifices.orifices.enum.spool_orifice.rectangle_slot  diameter_hole=0.005 m  num_hole=4  width=orificeWidth mm  del_S_max="spoolTravel  mm"  S_min=-overlap mm  open_orientation=fluids.isothermal_liquid.valves_orifices.enum.spool_orientation.negative  clearance=radClearance mm  area_leak=1e-9 m^2  smoothing_factor=0
      settings: InternalSimscapePortConfiguration="{\"Bottom\":[],\"Left\":[{\"id\":\"A\",\"label\":\"A\",\"type\":\"foundation.isothermal_liquid.isothermal_liquid\"},{\"id\":\"S\",\"label\":\"S\",\"type\":\"input\"}],\"Right\":[{\"id\":\"B\",\"label\":\"B\",\"type\":\"foundation.isothermal_liquid.isothermal_liquid\"},{\"id\":\"F\",\"label\":\"F\",\"type\":\"output\"}],\"Top\":[]}"
  S : PMIOPort  Side=Left
  A : PMIOPort  Port=2  Side=Left
  B : PMIOPort  Port=3  Side=Right
  connections:
  Motion Sensor/RConn3 -- Orifice/LConn1 -- Spool Orifice Hydraulic Force/LConn2
  Hydraulic Force/LConn1 -- Motion Sensor/LConn1 -- S/RConn1
  Orifice/RConn1 -- Spool Orifice Hydraulic Force/LConn1
  Orifice/LConn2 -- A/RConn1
  MTRef Force/LConn1 -- Hydraulic Force/RConn2
  MTRef Sensor/LConn1 -- Motion Sensor/RConn1
  Spool Orifice Hydraulic Force/RConn2 -- Hydraulic Force/RConn1
  Spool Orifice Hydraulic Force/RConn1 -- B/RConn1

== system PositionControlServoValve/Position Control Servo Valve/Valve Body/Orifice BT ==
  Hydraulic Force : fl_lib/Mechanical/Mechanical Sources/Ideal Force Source  Tag=Factory Generic
  MTRef Force : fl_lib/Mechanical/Translational Elements/Mechanical Translational Reference  Tag=Factory Generic
  MTRef Sensor : fl_lib/Mechanical/Translational Elements/Mechanical Translational Reference  Tag=Factory Generic
  Motion Sensor : fl_lib/Mechanical/Mechanical Sensors/Ideal Translational Motion Sensor  Tag=Factory Generic  reference=foundation.enum.MeasurementReference.difference  acceleration_port=false  velocity_port=true  position_port=true  offset=0 m
  Orifice : SimscapeFluids_lib/Isothermal Liquid/Valves & Orifices/Orifices/Spool Orifice (IL)  Tag=Factory Generic  orifice_spec=fluids.isothermal_liquid.valves_orifices.orifices.enum.spool_orifice.rectangle_slot  diameter_hole=5e-3 m  num_hole=6  width=orificeWidth mm  del_S_max="spoolTravel  mm"  S_min=overlap mm  open_orientation=fluids.isothermal_liquid.valves_orifices.enum.spool_orientation.positive  flow_force_spec=simscape.enum.onoff.off  clearance=1e-5 m  area_leak=1e-9 m^2  area=inf m^2  Cd=0.7  Re_c=150  smoothing_factor=0  pressure_recovery=simscape.enum.onoff.off
      settings: InternalSimscapePortConfiguration="{\"Bottom\":[],\"Left\":[{\"id\":\"S\",\"label\":\"S\",\"type\":\"input\"},{\"id\":\"A\",\"label\":\"A\",\"type\":\"foundation.isothermal_liquid.isothermal_liquid\"}],\"Right\":[{\"id\":\"B\",\"label\":\"B\",\"type\":\"foundation.isothermal_liquid.isothermal_liquid\"}],\"Top\":[]}"
  Spool Orifice Hydraulic Force : SimscapeFluids_lib/Isothermal Liquid/Valves & Orifices/Valve Actuators & Forces/Spool Orifice Flow Force (IL)  orifice_spec=fluids.isothermal_liquid.valves_orifices.orifices.enum.spool_orifice.rectangle_slot  diameter_hole=0.005 m  num_hole=4  width=orificeWidth mm  del_S_max="spoolTravel  mm"  S_min=overlap mm  open_orientation=fluids.isothermal_liquid.valves_orifices.enum.spool_orientation.positive  clearance=radClearance mm  area_leak=1e-9 m^2  smoothing_factor=0
      settings: InternalSimscapePortConfiguration="{\"Bottom\":[],\"Left\":[{\"id\":\"A\",\"label\":\"A\",\"type\":\"foundation.isothermal_liquid.isothermal_liquid\"},{\"id\":\"S\",\"label\":\"S\",\"type\":\"input\"}],\"Right\":[{\"id\":\"B\",\"label\":\"B\",\"type\":\"foundation.isothermal_liquid.isothermal_liquid\"},{\"id\":\"F\",\"label\":\"F\",\"type\":\"output\"}],\"Top\":[]}"
  S : PMIOPort  Side=Left
  A : PMIOPort  Port=2  Side=Left
  B : PMIOPort  Port=3  Side=Right
  connections:
  Motion Sensor/RConn3 -- Orifice/LConn1 -- Spool Orifice Hydraulic Force/LConn2
  Hydraulic Force/LConn1 -- Motion Sensor/LConn1 -- S/RConn1
  MTRef Sensor/LConn1 -- Motion Sensor/RConn1
  Orifice/LConn2 -- A/RConn1
  MTRef Force/LConn1 -- Hydraulic Force/RConn2
  Spool Orifice Hydraulic Force/RConn1 -- B/RConn1
  Spool Orifice Hydraulic Force/RConn2 -- Hydraulic Force/RConn1
  Orifice/RConn1 -- Spool Orifice Hydraulic Force/LConn1

== system PositionControlServoValve/Position Control Servo Valve/Valve Body/Orifice PA ==
  Hydraulic Force : fl_lib/Mechanical/Mechanical Sources/Ideal Force Source  Tag=Factory Generic
  MTRef Force : fl_lib/Mechanical/Translational Elements/Mechanical Translational Reference  Tag=Factory Generic
  MTRef Sensor : fl_lib/Mechanical/Translational Elements/Mechanical Translational Reference  Tag=Factory Generic
  Motion Sensor : fl_lib/Mechanical/Mechanical Sensors/Ideal Translational Motion Sensor  Tag=Factory Generic  reference=foundation.enum.MeasurementReference.difference  acceleration_port=false  velocity_port=true  position_port=true  offset=0 m
  Orifice : SimscapeFluids_lib/Isothermal Liquid/Valves & Orifices/Orifices/Spool Orifice (IL)  Tag=Factory Generic  orifice_spec=fluids.isothermal_liquid.valves_orifices.orifices.enum.spool_orifice.rectangle_slot  diameter_hole=5e-3 m  num_hole=6  width=orificeWidth mm  del_S_max="spoolTravel  mm"  S_min=overlap mm  open_orientation=fluids.isothermal_liquid.valves_orifices.enum.spool_orientation.positive  flow_force_spec=simscape.enum.onoff.off  clearance=1e-5 m  area_leak=1e-9 m^2  area=inf m^2  Cd=0.7  Re_c=150  smoothing_factor=0  pressure_recovery=simscape.enum.onoff.off
      settings: InternalSimscapePortConfiguration="{\"Bottom\":[],\"Left\":[{\"id\":\"S\",\"label\":\"S\",\"type\":\"input\"},{\"id\":\"A\",\"label\":\"A\",\"type\":\"foundation.isothermal_liquid.isothermal_liquid\"}],\"Right\":[{\"id\":\"B\",\"label\":\"B\",\"type\":\"foundation.isothermal_liquid.isothermal_liquid\"}],\"Top\":[]}"
  Spool Orifice Hydraulic Force : SimscapeFluids_lib/Isothermal Liquid/Valves & Orifices/Valve Actuators & Forces/Spool Orifice Flow Force (IL)  orifice_spec=fluids.isothermal_liquid.valves_orifices.orifices.enum.spool_orifice.rectangle_slot  diameter_hole=0.005 m  num_hole=4  width=orificeWidth mm  del_S_max="spoolTravel  mm"  S_min=overlap mm  open_orientation=fluids.isothermal_liquid.valves_orifices.enum.spool_orientation.positive  clearance=radClearance mm  area_leak=1e-9 m^2  smoothing_factor=0
      settings: InternalSimscapePortConfiguration="{\"Bottom\":[],\"Left\":[{\"id\":\"A\",\"label\":\"A\",\"type\":\"foundation.isothermal_liquid.isothermal_liquid\"},{\"id\":\"S\",\"label\":\"S\",\"type\":\"input\"}],\"Right\":[{\"id\":\"B\",\"label\":\"B\",\"type\":\"foundation.isothermal_liquid.isothermal_liquid\"},{\"id\":\"F\",\"label\":\"F\",\"type\":\"output\"}],\"Top\":[]}"
  S : PMIOPort  Side=Left
  A : PMIOPort  Port=2  Side=Left
  B : PMIOPort  Port=3  Side=Right
  connections:
  Spool Orifice Hydraulic Force/RConn2 -- Hydraulic Force/RConn1
  Spool Orifice Hydraulic Force/LConn1 -- Orifice/RConn1
  A/RConn1 -- Orifice/LConn2
  Spool Orifice Hydraulic Force/RConn1 -- B/RConn1
  Spool Orifice Hydraulic Force/LConn2 -- Motion Sensor/RConn3 -- Orifice/LConn1
  MTRef Sensor/LConn1 -- Motion Sensor/RConn1
  MTRef Force/LConn1 -- Hydraulic Force/RConn2
  S/RConn1 -- Motion Sensor/LConn1 -- Hydraulic Force/LConn1

== system PositionControlServoValve/Position Control Servo Valve/Valve Body/Orifice PB ==
  Hydraulic Force : fl_lib/Mechanical/Mechanical Sources/Ideal Force Source  Tag=Factory Generic
  MTRef Force : fl_lib/Mechanical/Translational Elements/Mechanical Translational Reference  Tag=Factory Generic
  MTRef Sensor : fl_lib/Mechanical/Translational Elements/Mechanical Translational Reference  Tag=Factory Generic
  Motion Sensor : fl_lib/Mechanical/Mechanical Sensors/Ideal Translational Motion Sensor  Tag=Factory Generic  reference=foundation.enum.MeasurementReference.difference  acceleration_port=false  velocity_port=true  position_port=true  offset=0 m
  Orifice : SimscapeFluids_lib/Isothermal Liquid/Valves & Orifices/Orifices/Spool Orifice (IL)  Tag=Factory Generic  orifice_spec=fluids.isothermal_liquid.valves_orifices.orifices.enum.spool_orifice.rectangle_slot  diameter_hole=5e-3 m  num_hole=6  width=orificeWidth mm  del_S_max="spoolTravel  mm"  S_min=-overlap mm  open_orientation=fluids.isothermal_liquid.valves_orifices.enum.spool_orientation.negative  flow_force_spec=simscape.enum.onoff.off  clearance=1e-5 m  area_leak=1e-9 m^2  area=inf m^2  Cd=0.7  Re_c=150  smoothing_factor=0  pressure_recovery=simscape.enum.onoff.off
      settings: InternalSimscapePortConfiguration="{\"Bottom\":[],\"Left\":[{\"id\":\"S\",\"label\":\"S\",\"type\":\"input\"},{\"id\":\"A\",\"label\":\"A\",\"type\":\"foundation.isothermal_liquid.isothermal_liquid\"}],\"Right\":[{\"id\":\"B\",\"label\":\"B\",\"type\":\"foundation.isothermal_liquid.isothermal_liquid\"}],\"Top\":[]}"
  Spool Orifice Hydraulic Force : SimscapeFluids_lib/Isothermal Liquid/Valves & Orifices/Valve Actuators & Forces/Spool Orifice Flow Force (IL)  orifice_spec=fluids.isothermal_liquid.valves_orifices.orifices.enum.spool_orifice.rectangle_slot  diameter_hole=0.005 m  num_hole=4  width=orificeWidth mm  del_S_max="spoolTravel  mm"  S_min=-overlap mm  open_orientation=fluids.isothermal_liquid.valves_orifices.enum.spool_orientation.negative  clearance=radClearance mm  area_leak=1e-9 m^2  smoothing_factor=0
      settings: InternalSimscapePortConfiguration="{\"Bottom\":[],\"Left\":[{\"id\":\"A\",\"label\":\"A\",\"type\":\"foundation.isothermal_liquid.isothermal_liquid\"},{\"id\":\"S\",\"label\":\"S\",\"type\":\"input\"}],\"Right\":[{\"id\":\"B\",\"label\":\"B\",\"type\":\"foundation.isothermal_liquid.isothermal_liquid\"},{\"id\":\"F\",\"label\":\"F\",\"type\":\"output\"}],\"Top\":[]}"
  S : PMIOPort  Side=Left
  A : PMIOPort  Port=2  Side=Left
  B : PMIOPort  Port=3  Side=Right
  connections:
  Motion Sensor/RConn3 -- Orifice/LConn1 -- Spool Orifice Hydraulic Force/LConn2
  S/RConn1 -- Motion Sensor/LConn1 -- Hydraulic Force/LConn1
  Spool Orifice Hydraulic Force/RConn2 -- Hydraulic Force/RConn1
  Orifice/LConn2 -- A/RConn1
  MTRef Force/LConn1 -- Hydraulic Force/RConn2
  MTRef Sensor/LConn1 -- Motion Sensor/RConn1
  Orifice/RConn1 -- Spool Orifice Hydraulic Force/LConn1
  Spool Orifice Hydraulic Force/RConn1 -- B/RConn1

== system PositionControlServoValve/Position Control Servo Valve/Valve Body1/Orifice AT ==
  Hydraulic Force : fl_lib/Mechanical/Mechanical Sources/Ideal Force Source  Tag=Factory Generic
  MTRef Force : fl_lib/Mechanical/Translational Elements/Mechanical Translational Reference  Tag=Factory Generic
  MTRef Sensor : fl_lib/Mechanical/Translational Elements/Mechanical Translational Reference  Tag=Factory Generic
  Motion Sensor : fl_lib/Mechanical/Mechanical Sensors/Ideal Translational Motion Sensor  Tag=Factory Generic  reference=foundation.enum.MeasurementReference.difference  acceleration_port=false  velocity_port=true  position_port=true  offset=0 m
  Orifice : SimscapeFluids_lib/Isothermal Liquid/Valves & Orifices/Orifices/Spool Orifice (IL)  Tag=Factory Generic  orifice_spec=fluids.isothermal_liquid.valves_orifices.orifices.enum.spool_orifice.rectangle_slot  diameter_hole=5e-3 m  num_hole=6  width=orificeWidth mm  del_S_max="spoolTravel  mm"  S_min=-overlap mm  open_orientation=fluids.isothermal_liquid.valves_orifices.enum.spool_orientation.negative  flow_force_spec=simscape.enum.onoff.off  clearance=1e-5 m  area_leak=1e-9 m^2  area=inf m^2  Cd=0.7  Re_c=150  smoothing_factor=0  pressure_recovery=simscape.enum.onoff.off
      settings: InternalSimscapePortConfiguration="{\"Bottom\":[],\"Left\":[{\"id\":\"S\",\"label\":\"S\",\"type\":\"input\"},{\"id\":\"A\",\"label\":\"A\",\"type\":\"foundation.isothermal_liquid.isothermal_liquid\"}],\"Right\":[{\"id\":\"B\",\"label\":\"B\",\"type\":\"foundation.isothermal_liquid.isothermal_liquid\"}],\"Top\":[]}"
  Spool Orifice Hydraulic Force : SimscapeFluids_lib/Isothermal Liquid/Valves & Orifices/Valve Actuators & Forces/Spool Orifice Flow Force (IL)  orifice_spec=fluids.isothermal_liquid.valves_orifices.orifices.enum.spool_orifice.rectangle_slot  diameter_hole=0.005 m  num_hole=4  width=orificeWidth mm  del_S_max="spoolTravel  mm"  S_min=-overlap mm  open_orientation=fluids.isothermal_liquid.valves_orifices.enum.spool_orientation.negative  clearance=radClearance mm  area_leak=1e-9 m^2  smoothing_factor=0
      settings: InternalSimscapePortConfiguration="{\"Bottom\":[],\"Left\":[{\"id\":\"A\",\"label\":\"A\",\"type\":\"foundation.isothermal_liquid.isothermal_liquid\"},{\"id\":\"S\",\"label\":\"S\",\"type\":\"input\"}],\"Right\":[{\"id\":\"B\",\"label\":\"B\",\"type\":\"foundation.isothermal_liquid.isothermal_liquid\"},{\"id\":\"F\",\"label\":\"F\",\"type\":\"output\"}],\"Top\":[]}"
  S : PMIOPort  Side=Left
  A : PMIOPort  Port=2  Side=Left
  B : PMIOPort  Port=3  Side=Right
  connections:
  Motion Sensor/RConn3 -- Orifice/LConn1 -- Spool Orifice Hydraulic Force/LConn2
  Hydraulic Force/LConn1 -- Motion Sensor/LConn1 -- S/RConn1
  Orifice/RConn1 -- Spool Orifice Hydraulic Force/LConn1
  Orifice/LConn2 -- A/RConn1
  MTRef Force/LConn1 -- Hydraulic Force/RConn2
  MTRef Sensor/LConn1 -- Motion Sensor/RConn1
  Spool Orifice Hydraulic Force/RConn2 -- Hydraulic Force/RConn1
  Spool Orifice Hydraulic Force/RConn1 -- B/RConn1
